simulink model "step_aprbs"  (R2014a)
settings: Solver=ode45  StartTime=0.0  StopTime=300  RelTol=1e-3
settings Model: Creator=Lab Automática  LastModifiedBy=Lab Automática

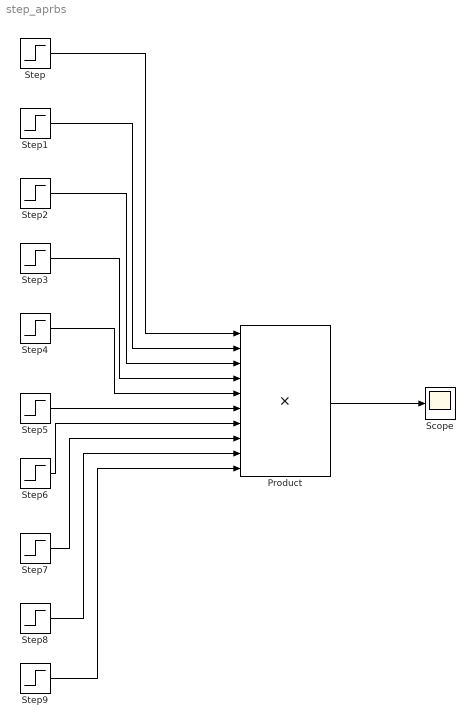
== system step_aprbs ==
  Product : Product  Inputs=10
  Scope : Scope
  Step : Step  Time=0  Before=10  SampleTime=0
  Step1 : Step  Time=30  Before=11.5  SampleTime=0
  Step2 : Step  Time=60  Before=13  SampleTime=0
  Step3 : Step  Time=90  Before=14.5  SampleTime=0
  Step4 : Step  Time=120  Before=16  SampleTime=0
  Step5 : Step  Time=150  Before=17.5  SampleTime=0
  Step6 : Step  Time=180  Before=19  SampleTime=0
  Step7 : Step  Time=210  Before=20.5  SampleTime=0
  Step8 : Step  Time=240  Before=22  SampleTime=0
  Step9 : Step  Time=270  Before=23.5  SampleTime=0
  wires:
  Step/1 -> Product/1
  Step1/1 -> Product/2
  Step2/1 -> Product/3
  Step3/1 -> Product/4
  Step4/1 -> Product/5
  Step5/1 -> Product/6
  Step6/1 -> Product/7
  Step7/1 -> Product/8
  Step8/1 -> Product/9
  Step9/1 -> Product/10
  Product/1 -> Scope/1
